simulink model "mpc555rt_led"  (Simulink 7.4)
settings: Solver=FixedStepDiscrete  StartTime=0.0  StopTime=inf  FixedStep=0.01  RelTol=1e-3
PreLoadFcn:
  | RTWConfigurationCB('preloadfcn', bdroot);
PostLoadFcn:
  | mpc555rt_switch_target(gcs,'auto')
libraries: mpc555drivers x3, pil_demo_lib x1
CloseFcn:
  | rtwprivate ssgencode ModelCloseRequest foo
settings Model: Creator=The MathWorks Inc.  LastModifiedBy=autopilot
settings DataIOCC: SignalLoggingName=sigsOut
settings OptimizationCC: InlineParams=on  InlineInvariantSignals=on  EnforceIntegerDowncast=off  ZeroExternalMemoryAtStartup=off  ZeroInternalMemoryAtStartup=off  InitFltsAndDblsToZero=on  NoFixptDivByZeroProtection=on  OptimizeModelRefInitCode=on  LifeSpan=1
settings DebuggingCC: SaveWithParameterizedLinksMsg=none  SignalResolutionControl=TryResolveAllWithWarning  SolverPrmCheckMsg=none  MultiTaskDSMMsg=warning  MultiTaskCondExecSysMsg=none  UnderSpecifiedDataTypeMsg=error  StrictBusMsg=None
settings HardwareCC: ProdEndianess=BigEndian  ProdHWDeviceType=Motorola PowerPC
settings RTWCC: SystemTargetFile=mpc555rt.tlc  TemplateMakefile=mpc555rt.tmf  Description=Target Support Package (for use with Freescale MPC5xx) (real-time)  ProcessScript=mpc555rt_make_rtw_hook
settings CodeAppCC: IgnoreCustomStorageClasses=off
settings STFCustomTargetCC: TargetFcnLib=ansi_tfl_tmw.mat  TargetLibSuffix=.a  TargetPreCompLibLocation=C:\Program Files\MATLAB\R2009b\toolbox\rtw\targets\mpc555dk\drivers\lib\DIAB  IncludeMdlTerminateFcn=off  CombineOutputUpdateFcns=on  ERTCustomFileBanners=on  SupportAbsoluteTime=off  SupportNonFinite=off  SupportComplex=off  SupportContinuousTime=off  SupportNonInlinedSFcns=off  CPPClassGenCompliant=on  SystemTargetFile=mpc555rt.tlc
settings ERTTargetCC: TargetFcnLib=ansi_tfl_tmw.mat  TargetPreCompLibLocation=C:\Program Files\MATLAB\R2009b\toolbox\rtw\targets\mpc555dk\drivers\lib\DIAB  MultiwordLength=2048  ParMdlRefBuildCompliant=off  CompOptLevelCompliant=off  IncludeMdlTerminateFcn=off  ERTFirstTimeCompliant=off  SupportAbsoluteTime=off  SupportNonFinite=off  SupportComplex=off  ModelStepFunctionPrototypeControlCompliant=off  ExtModeMexFile=MPC5xxExternalModeOpen  ExtModeIntrfLevel=Level2 - Open  ERTCustomFileTemplate=example_file_process.tlc  ConvertIfToSwitch=off
settings CustomProperty: DataType=RTWOptions_EnumType__toolbox_rtw_targets_mpc555dk_mpc555dk_mpc555rt_1MPC555_OPTIMIZATION_SWITCH  Value=speed
settings EnumStrPairs: String=speed

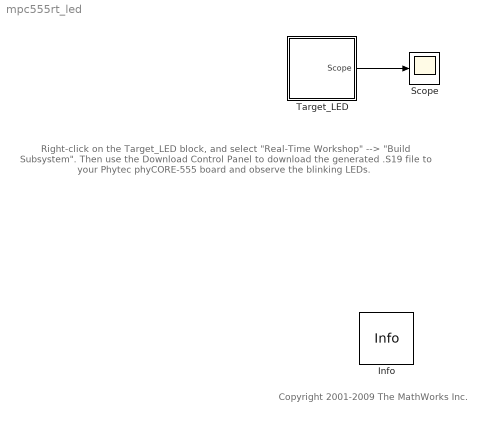
== system mpc555rt_led ==
  note: Right-click on the Target_LED block, and select
      | "Real-Time Workshop" --> "Build Subsystem".
      | Then use the Download Control Panel to
      | download the generated .S19 file to your
      | Phytec phyCORE-555 board and observe the
      | blinking LEDs.
  note: Copyright 2001-2009 The MathWorks Inc.
  Info : pil_demo_lib/Info  SystemSampleTime=-1
  Scope : Scope
      settings: YMin=0  YMax=1
  Target_LED : Subsystem  InitFcn=|
      | % START RTW CONFIGURATION CODE %
      | RTWConfigurationCB('rtw_target_initfcn',gcb);
      | % END RTW CONFIGURATION CODE %
      mask Display: image(imread('target_affordance_icon.jpg'),'bottom-right')
  wires:
  Target_LED/1(Scope) -> Scope/1

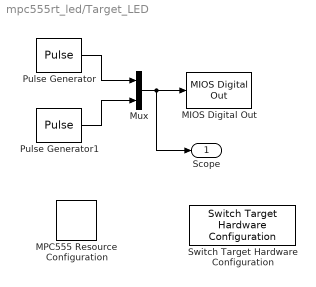
== system mpc555rt_led/Target_LED ==
  MIOS Digital Out : mpc555drivers/Modular Input//Output System (MIOS1)/MIOS Digital Out  SystemSampleTime=-1  bits=[0 1]  init=0  t=-1  enablePassThru=off
  MPC555 Resource Configuration : mpc555drivers/MPC555 Resource Configuration  Tag=RTW CONFIGURATION BLOCK  Priority=-100000  SystemSampleTime=-1  oldParentName=mpc555rt_led/Target_LED  oldBlockName=|  defaultConfigLibrary=mpc555drivers
      | mpc555rt_led/Target_LED/MPC555
      | Resource
      | Configuration
  Mux : Mux  Inputs=2
  Pulse Generator : DiscretePulseGenerator  Amplitude=1  Period=100  PulseWidth=50  PhaseDelay=0  SampleTime=0.01  VectorParams1D=off
  Pulse Generator1 : DiscretePulseGenerator  Amplitude=1  Period=50  PulseWidth=25  PhaseDelay=0  SampleTime=0.01
  Switch Target Hardware Configuration : mpc555drivers/Utilities/Switch Target Hardware Configuration  SystemSampleTime=-1
  Scope : Outport  OutDataType=sfix(16)  OutScaling=2^0
  wires:
  Mux/1 -> MIOS Digital Out/1, Scope/1
  Pulse Generator/1 -> Mux/1
  Pulse Generator1/1 -> Mux/2
